simulink model "Plant_N_LQR_Joystick"  (R2017a)
settings: Solver=ode5  StartTime=0.0  StopTime=100  FixedStep=0.001  RelTol=1e-3  EnableMultiTasking=on
InitFcn:
  | close all;
values from neighbouring files (symbols this model uses):
  K_LQR = -R1\B'*P    [Sc_H2LQR_R.m]
libraries: aerolibanimutils x2
settings Model: Creator=GeoLee  LastModifiedBy=gmh_n
settings DataIOCC: LimitDataPoints=on  SaveFormat=Array  SaveOutput=off  SignalLogging=off  DSMLogging=off  SaveTime=off
settings OptimizationCC: LifeSpan=inf
settings DebuggingCC: SFUnexpectedBacktrackingDiag=warning  SFNoUnconditionalDefaultTransitionDiag=warning  SFExecutionAtInitializationDiag=none
settings HardwareCC: ProdBitPerPointer=32  ProdBitPerSizeT=32  ProdBitPerPtrDiffT=32  ProdLargestAtomicFloat=None  ProdIntDivRoundTo=Undefined  ProdEndianess=Unspecified  ProdWordSize=32  ProdHWDeviceType=32-bit Generic
settings ModelReferenceCC: PropagateSignalLabelsOutOfModel=off
settings GRTTargetCC: TargetLangStandard=C89/C90 (ANSI)  GeneratePreprocessorConditionals=Disable all
settings ConfigComp: CovMetricSettings=dw  CovHtmlReporting=on  CovSaveCumulativeToWorkspaceVar=on  CovSaveSingleToWorkspaceVar=on  CovExternalEMLEnable=off

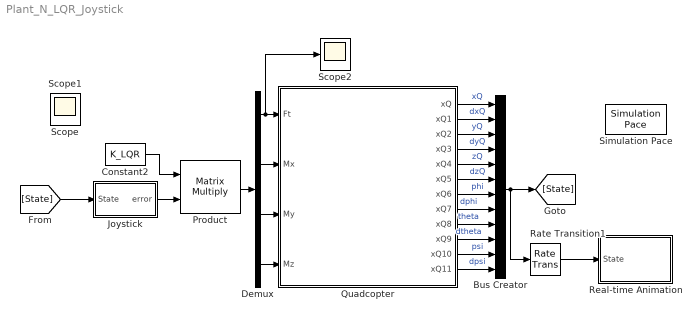
== system Plant_N_LQR_Joystick ==
  Bus Creator : BusCreator  Inputs=12
  Constant2 : Constant  Value=K_LQR
  Demux : Demux
  Joystick : Subsystem
  Product : Product  Multiplication=Matrix(*)  RndMeth=Zero
  Quadcopter : Subsystem  mask(Single Quadcopter Plant){x0=0, y0=0, z0=0}
      mask prompts: x0 "Initial position of x (m)"; y0 "Initial position of y (m)"; z0 "Initial position of z (m)"
      mask help:
      | Attention:
      | the first input Ft is actually dF!
      mask Display:
      | image('Quad_pic.png');
      | port_label('input', 1, 'Ft');
      | port_label('input', 2, 'Mx');
      | port_label('input', 3, 'My');
      | port_label('input', 4, 'Mz');
      | port_label('output', 1, 'xQ');
      | port_label('output', 2, 'dxQ');
      | port_label('output', 3, 'yQ');
      | port_label('output', 4, 'dyQ');
      | port_label('output', 5, 'zQ');
      | port_label('output', 6, 'dzQ');
      | port_label('output', 7, 'phi');
      | port_label('output', 8, 'dphi');
      | port_label('output', 9, 'theta');
      | port_label('output', 10, 'dtheta');
      | port_label('output', 11, 'psi');
      | port_label('output', 12, 'dpsi');
  Rate Transition1 : RateTransition  OutPortSampleTime=0.05
  Real-time Animation : Stateflow chart  TreatAsAtomicUnit=on
  Scope2 : Scope
  Simulation Pace : aerolibanimutils/Simulation Pace  SimulationPace=1  SleepMode=MATLAB Thread  OutputPaceError=off  SampleTime=-1
  Scope : Scope
  Scope1 : Scope
  wires:
  Product/1 -> Demux/1
  [State] -> Joystick/1(State)
  Joystick/1(error) -> Product/2
  Quadcopter/6(xQ5) -> Bus Creator/6  "dzQ"
  Quadcopter/5(xQ4) -> Bus Creator/5  "zQ"
  Quadcopter/7(xQ6) -> Bus Creator/7  "phi"
  Quadcopter/4(xQ3) -> Bus Creator/4  "dyQ"
  Quadcopter/8(xQ7) -> Bus Creator/8  "dphi"
  Quadcopter/3(xQ2) -> Bus Creator/3  "yQ"
  Quadcopter/9(xQ8) -> Bus Creator/9  "theta"
  Quadcopter/2(xQ1) -> Bus Creator/2  "dxQ"
  Quadcopter/10(xQ9) -> Bus Creator/10  "dtheta"
  Quadcopter/11(xQ10) -> Bus Creator/11  "psi"
  Quadcopter/1(xQ) -> Bus Creator/1  "xQ"
  Quadcopter/12(xQ11) -> Bus Creator/12  "dpsi"
  Demux/2 -> Quadcopter/2(Mx)
  Demux/4 -> Quadcopter/4(Mz)
  Demux/3 -> Quadcopter/3(My)
  Constant2/1 -> Product/1
  Demux/1 -> Scope2/1, Quadcopter/1(Ft)
  Bus Creator/1 -> Rate Transition1/1, [State]
  Rate Transition1/1 -> Real-time Animation/1(State)

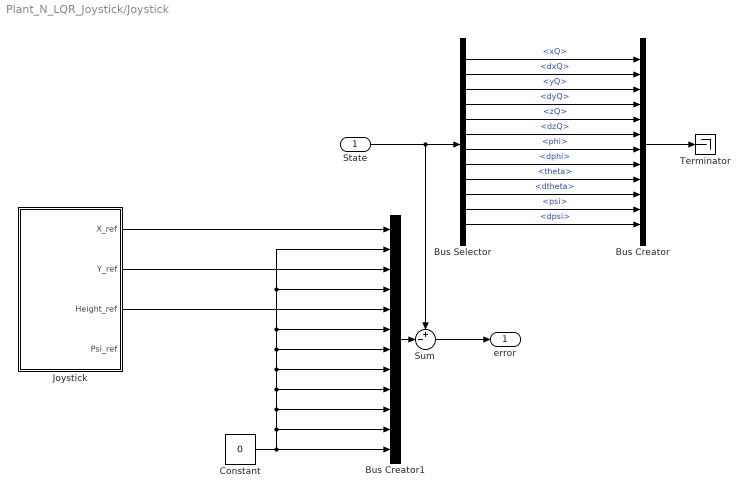
== system Plant_N_LQR_Joystick/Joystick ==
  State : Inport
  Bus Creator : BusCreator  Inputs=12
  Bus Creator1 : BusCreator  Inputs=12
  Bus Selector : BusSelector  OutputSignals=xQ,dxQ,yQ,dyQ,zQ,dzQ,phi,dphi,theta,dtheta,psi,dpsi
  Constant : Constant  Value=0
  Joystick : Subsystem
  Sum : Sum  Inputs=+-|
  Terminator : Terminator
  error : Outport
  wires:
  Bus Selector/3 -> Bus Creator/3  "<yQ>"
  Bus Selector/9 -> Bus Creator/9  "<theta>"
  Bus Selector/10 -> Bus Creator/10  "<dtheta>"
  Bus Selector/7 -> Bus Creator/7  "<phi>"
  Bus Selector/2 -> Bus Creator/2  "<dxQ>"
  Bus Selector/8 -> Bus Creator/8  "<dphi>"
  Bus Selector/5 -> Bus Creator/5  "<zQ>"
  Bus Selector/4 -> Bus Creator/4  "<dyQ>"
  Bus Selector/11 -> Bus Creator/11  "<psi>"
  Bus Creator/1 -> Terminator/1
  Bus Selector/12 -> Bus Creator/12  "<dpsi>"
  Bus Selector/1 -> Bus Creator/1  "<xQ>"
  State/1 -> Bus Selector/1, Sum/1
  Bus Selector/6 -> Bus Creator/6  "<dzQ>"
  Bus Creator1/1 -> Sum/2
  Sum/1 -> error/1
  Constant/1 -> Bus Creator1/11, Bus Creator1/10, Bus Creator1/9, Bus Creator1/8, Bus Creator1/7, Bus Creator1/6, Bus Creator1/4, Bus Creator1/2, Bus Creator1/12
  Joystick/1(X_ref) -> Bus Creator1/1
  Joystick/2(Y_ref) -> Bus Creator1/3
  Joystick/3(Height_ref) -> Bus Creator1/5

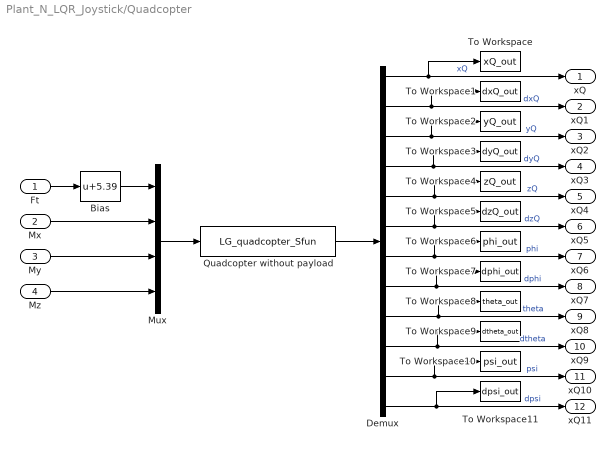
== system Plant_N_LQR_Joystick/Quadcopter ==
  Ft : Inport
  Mx : Inport  Port=2
  My : Inport  Port=3
  Mz : Inport  Port=4
  Bias : Bias  Bias=5.39
  Demux : Demux  Outputs=12
  Mux : Mux
  Quadcopter without payload : S-Function  FunctionName=LG_quadcopter_Sfun  Parameters=x0,y0,z0  SFunctionDeploymentMode=off  EnableBusSupport=off
  To Workspace : ToWorkspace  VariableName=xQ_out  SampleTime=-1
  To Workspace1 : ToWorkspace  VariableName=dxQ_out  SampleTime=-1
  To Workspace10 : ToWorkspace  VariableName=psi_out  SampleTime=-1
  To Workspace11 : ToWorkspace  VariableName=dpsi_out  SampleTime=-1
  To Workspace2 : ToWorkspace  VariableName=yQ_out  SampleTime=-1
  To Workspace3 : ToWorkspace  VariableName=dyQ_out  SampleTime=-1
  To Workspace4 : ToWorkspace  VariableName=zQ_out  SampleTime=-1
  To Workspace5 : ToWorkspace  VariableName=dzQ_out  SampleTime=-1
  To Workspace6 : ToWorkspace  VariableName=phi_out  SampleTime=-1
  To Workspace7 : ToWorkspace  VariableName=dphi_out  SampleTime=-1
  To Workspace8 : ToWorkspace  VariableName=theta_out  SampleTime=-1
  To Workspace9 : ToWorkspace  VariableName=dtheta_out  SampleTime=-1
  xQ : Outport
  xQ1 : Outport  Port=2
  xQ2 : Outport  Port=3
  xQ3 : Outport  Port=4
  xQ4 : Outport  Port=5
  xQ5 : Outport  Port=6
  xQ6 : Outport  Port=7
  xQ7 : Outport  Port=8
  xQ8 : Outport  Port=9
  xQ9 : Outport  Port=10
  xQ10 : Outport  Port=11
  xQ11 : Outport  Port=12
  wires:
  Mux/1 -> Quadcopter without payload/1
  Ft/1 -> Bias/1
  Quadcopter without payload/1 -> Demux/1
  Mz/1 -> Mux/4
  Bias/1 -> Mux/1
  Demux/9 -> To Workspace8/1, xQ8/1  "theta"
  Demux/1 -> xQ/1, To Workspace/1  "xQ"
  Demux/7 -> xQ6/1, To Workspace6/1  "phi"
  Demux/11 -> xQ10/1, To Workspace10/1  "psi"
  Demux/4 -> xQ3/1, To Workspace3/1  "dyQ"
  Demux/2 -> xQ1/1, To Workspace1/1  "dxQ"
  Demux/3 -> xQ2/1, To Workspace2/1  "yQ"
  Demux/10 -> xQ9/1, To Workspace9/1  "dtheta"
  Demux/5 -> xQ4/1, To Workspace4/1  "zQ"
  Demux/8 -> xQ7/1, To Workspace7/1  "dphi"
  Demux/12 -> xQ11/1, To Workspace11/1  "dpsi"
  Demux/6 -> xQ5/1, To Workspace5/1  "dzQ"
  My/1 -> Mux/3
  Mx/1 -> Mux/2

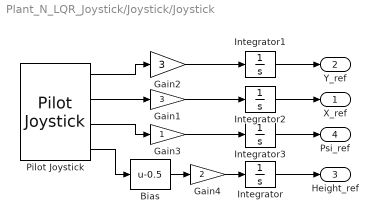
== system Plant_N_LQR_Joystick/Joystick/Joystick ==
  Bias : Bias  Bias=-0.5
  Gain1 : Gain  Gain=3
  Gain2 : Gain  Gain=3
  Gain3 : Gain
  Gain4 : Gain  Gain=2
  Integrator{,1..3} (4 alike) : Integrator
  Pilot Joystick : aerolibanimutils/Pilot Joystick  JoystickID=Joystick1  OutputConfiguration=FourAxis  SampleTime=0.001
  X_ref : Outport
  Y_ref : Outport  Port=2
  Height_ref : Outport  Port=3
  Psi_ref : Outport  Port=4
  wires:
  Gain3/1 -> Integrator3/1
  Pilot Joystick/4 -> Bias/1
  Bias/1 -> Gain4/1
  Pilot Joystick/3 -> Gain3/1
  Pilot Joystick/1 -> Gain2/1
  Pilot Joystick/2 -> Gain1/1
  Integrator/1 -> Height_ref/1
  Gain2/1 -> Integrator1/1
  Gain1/1 -> Integrator2/1
  Integrator3/1 -> Psi_ref/1
  Integrator1/1 -> Y_ref/1
  Integrator2/1 -> X_ref/1
  Gain4/1 -> Integrator/1

== stateflow chart Plant_N_LQR_Joystick/Real-time Animation ==
  settings: sampleTime=0.01
  state Plot
    entry:
    fig = ml.figure();
    phandles = ml.LG_plot_initial(fig,State);
    du:
    ml.LG_plot_update(fig,State,phandles);
  (default) -> Plot
  data: State input double size=12; fig local ml; phandles local ml
